simulink model "ground_control_station"  (R2022a)
settings: Solver=VariableStepAuto  StartTime=0.0  StopTime=10.0  RelTol=1e-3
undefined symbols (not defined in the file): CR, LF
libraries: instrumentseriallib x2
settings Model: Creator=kavin  LastModifiedBy=kavin

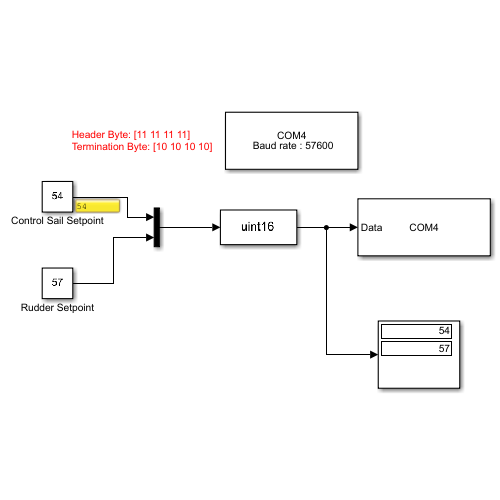
[thumbnail: Simulink's stored preview of the top-level diagram]
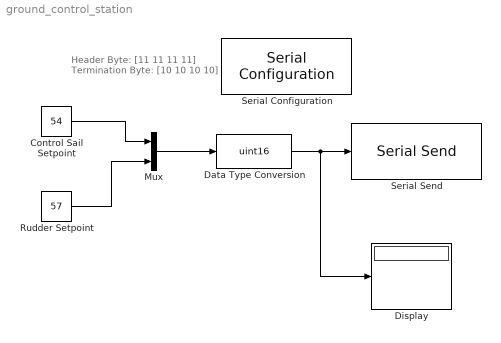
== system ground_control_station ==
  note: Header Byte: [11 11 11 11]
      | Termination Byte: [10 10 10 10]
  Control Sail Setpoint : Constant  Value=54  SampleTime=-1
  Data Type Conversion : DataTypeConversion  OutDataTypeStr=uint16  SaturateOnIntegerOverflow=off  RndMeth=Floor
  Display : Display
  Mux : Mux  Inputs=2
  Rudder Setpoint : Constant  Value=57
  Serial Configuration : instrumentseriallib/Serial Configuration  Priority=-200000  PortSel=COM4  Port=COM4  ComPort=COM4  BaudRate=57600  DataBits=8  Parity=none  StopBits=1  ByteOrder=little-endian  FlowControl=none  Timeout=10  SimulateUsing=Interpreted execution  BlockInModel=on  aMode=1
      settings: SourceProductBaseCode=OT,IC,MT
  Serial Send : instrumentseriallib/Serial Send  Priority=1  PortSel=COM4  Port=COM4  ComPort=COM4  Header=[11 11 11 11]  Terminator=CR/LF ('\r\n')  CustomTerminator=[10 10 10 10]  EnableBlockingMode=on  SimulateUsing=Interpreted execution  BlockInModel=on  aMode=1
      settings: SourceProductBaseCode=OT,IC,MT
  wires:
  Control Sail Setpoint/1 -> Mux/1
  Rudder Setpoint/1 -> Mux/2
  Mux/1 -> Data Type Conversion/1
  Data Type Conversion/1 -> Display/1, Serial Send/1
